simulink model "P71s"  (R2015b)
settings: Solver=VariableStepAuto  StartTime=0.0  StopTime=10.0  RelTol=1e-3
settings Model: Creator=xmax1946  LastModifiedBy=xmax1946

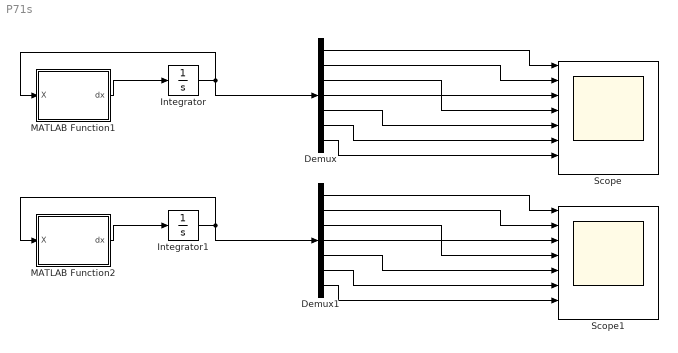
== system P71s ==
  Demux : Demux  Outputs=7
  Demux1 : Demux  Outputs=7
  Integrator : Integrator  InitialCondition=[0;0;1;1;1;0;0]
  Integrator1 : Integrator  InitialCondition=[0;0;1;1;1;0;0]
  MATLAB Function1 : MATLAB Function  TreatAsAtomicUnit=on
  MATLAB Function2 : MATLAB Function  TreatAsAtomicUnit=on
  Scope : Scope  NumInputPorts=8
  Scope1 : Scope  NumInputPorts=8
  wires:
  MATLAB Function1/1(dx) -> Integrator/1
  Integrator/1 -> Demux/1, MATLAB Function1/1(X)
  Demux/1 -> Scope/1
  Demux/2 -> Scope/2
  Demux/3 -> Scope/3
  Demux/4 -> Scope/4
  Demux/5 -> Scope/5
  Demux/6 -> Scope/6
  Demux/7 -> Scope/7
  MATLAB Function2/1(dx) -> Integrator1/1
  Integrator1/1 -> Demux1/1, MATLAB Function2/1(X)
  Demux1/1 -> Scope1/1
  Demux1/2 -> Scope1/2
  Demux1/3 -> Scope1/3
  Demux1/4 -> Scope1/4
  Demux1/5 -> Scope1/5
  Demux1/6 -> Scope1/6
  Demux1/7 -> Scope1/7

== matlab function P71s/MATLAB Function1 ==
  data: dx output; X input
function dx  = fcn(X)
A=[-5,6,-6,11,-8,-1,2
    -3,1,-3,4,-5,-1,6
    0,0,-5,11,-14,-1,8
    0,0,-8,14,-14,8,-5
    0,0,-8,15,-8,8,-12
    0,0,-8,8,0,2,-7
    0,0,-8,8,0,8,-13];
B=[3;2;1;0;0;1;0];
K=[4139/150,-2831/75,-751/30,4139/150,-3267/50,2831/75,6778/75];
u=1-K*X;
dx=A*X+B*u;

== matlab function P71s/MATLAB Function2 ==
  data: dx output; X input
function dx  = fcn(X)
A=[-5,6,-6,11,-8,-1,2
    -3,1,-3,4,-5,-1,6
    0,0,-5,11,-14,-1,8
    0,0,-8,14,-14,8,-5
    0,0,-8,15,-8,8,-12
    0,0,-8,8,0,2,-7
    0,0,-8,8,0,8,-13];
B=[3;2;1;0;0;1;0];
u=1;
dx=A*X+B*u;
